simulink model "Microstick_II_CodeReplacementLookup_ExternalMode_R2016b"  (R2016b)
settings: Solver=FixedStepDiscrete  StartTime=0.0  StopTime=inf  FixedStep=0.01  RelTol=1e-3
undefined symbols (not defined in the file or in its folder): A4, B0, B10, B11, B12, Max, MaxPer, ms, P20, P32, P42, P43, Pin, Resol, us
libraries: MCHP_Blockset x10
(part 2 of 2)

== system Microstick_II_CodeReplacementLookup_ExternalMode_R2016b/Cos/Cos Q15 ==
  In2 : Inport
  MCHP_Cos_Q1.15 : Subsystem  TreatAsAtomicUnit=on
  Cos_Out1 : Outport  OutDataTypeStr=fixdt(1,16,14)
  wires:
  In2/1 -> MCHP_Cos_Q1.15/1(In1)
  MCHP_Cos_Q1.15/1(Out1) -> Cos_Out1/1

== system Microstick_II_CodeReplacementLookup_ExternalMode_R2016b/Microstick2 - dsPIC33EP128MC202/1Hz Blinking2 ==
  Delay : Delay  DelayLength=1  InitialCondition=0  SampleTime=.5
  Logical Operator : Logic  Operator=NOT  AllPortsSameDT=off  OutDataTypeStr=boolean
  Rate Transition2 : RateTransition  Deterministic=off  OutPortSampleTime=.05
  Out1 : Outport
  wires:
  Delay/1 -> Logical Operator/1
  Logical Operator/1 -> Delay/1, Rate Transition2/1
  Rate Transition2/1 -> Out1/1

== system Microstick_II_CodeReplacementLookup_ExternalMode_R2016b/Microstick2 - dsPIC33EP128MC202/Open board doc WWW ==

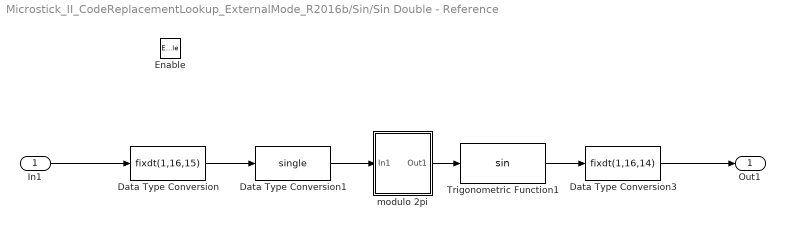
== system Microstick_II_CodeReplacementLookup_ExternalMode_R2016b/Sin/Sin Double - Reference ==
  In1 : Inport
  Enable : EnablePort
  Data Type Conversion : DataTypeConversion  OutDataTypeStr=fixdt(1,16,15)  ConvertRealWorld=Stored Integer (SI)
  Data Type Conversion1 : DataTypeConversion  OutDataTypeStr=single
  Data Type Conversion3 : DataTypeConversion  OutDataTypeStr=fixdt(1,16,14)  RndMeth=Convergent  SaturateOnIntegerOverflow=on
  Trigonometric Function1 : Trigonometry  NumberOfIterations=15
  modulo 2pi : Subsystem
  Out1 : Outport
  wires:
  Data Type Conversion3/1 -> Out1/1
  modulo 2pi/1(Out1) -> Trigonometric Function1/1
  Data Type Conversion1/1 -> modulo 2pi/1(In1)
  Data Type Conversion/1 -> Data Type Conversion1/1
  Trigonometric Function1/1 -> Data Type Conversion3/1
  In1/1 -> Data Type Conversion/1

== system Microstick_II_CodeReplacementLookup_ExternalMode_R2016b/Sin/Sin Q15 ==
  In2 : Inport
  MCHP_Sin_Q1.15 : Subsystem  TreatAsAtomicUnit=on
  Sin_Out1 : Outport  OutDataTypeStr=fixdt(1,16,14)
  wires:
  MCHP_Sin_Q1.15/1(Out1) -> Sin_Out1/1
  In2/1 -> MCHP_Sin_Q1.15/1(In1)

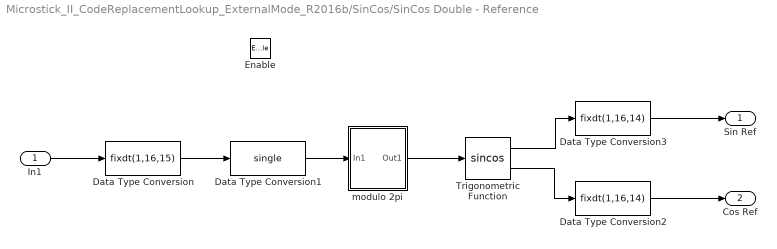
== system Microstick_II_CodeReplacementLookup_ExternalMode_R2016b/SinCos/SinCos Double - Reference ==
  In1 : Inport
  Enable : EnablePort
  Data Type Conversion : DataTypeConversion  OutDataTypeStr=fixdt(1,16,15)  ConvertRealWorld=Stored Integer (SI)
  Data Type Conversion1 : DataTypeConversion  OutDataTypeStr=single
  Data Type Conversion2 : DataTypeConversion  OutDataTypeStr=fixdt(1,16,14)  RndMeth=Convergent  SaturateOnIntegerOverflow=on
  Data Type Conversion3 : DataTypeConversion  OutDataTypeStr=fixdt(1,16,14)  RndMeth=Convergent  SaturateOnIntegerOverflow=on
  Trigonometric Function : Trigonometry  Operator=sincos
  modulo 2pi : Subsystem
  Sin Ref : Outport
  Cos Ref : Outport  Port=2
  wires:
  Data Type Conversion3/1 -> Sin Ref/1
  modulo 2pi/1(Out1) -> Trigonometric Function/1
  Data Type Conversion1/1 -> modulo 2pi/1(In1)
  Data Type Conversion/1 -> Data Type Conversion1/1
  Trigonometric Function/1 -> Data Type Conversion3/1
  In1/1 -> Data Type Conversion/1
  Data Type Conversion2/1 -> Cos Ref/1
  Trigonometric Function/2 -> Data Type Conversion2/1

== system Microstick_II_CodeReplacementLookup_ExternalMode_R2016b/SinCos/SinCos Q15 ==
  In2 : Inport
  MCHP_SinCos_Q1.15 : Subsystem  TreatAsAtomicUnit=on
  Sin_Out : Outport  OutDataTypeStr=fixdt(1,16,14)
  Cos_Out : Outport  Port=2  OutDataTypeStr=fixdt(1,16,14)
  wires:
  MCHP_SinCos_Q1.15/1(Out1) -> Sin_Out/1
  In2/1 -> MCHP_SinCos_Q1.15/1(In1)
  MCHP_SinCos_Q1.15/2(Out2) -> Cos_Out/1

== system Microstick_II_CodeReplacementLookup_ExternalMode_R2016b/Sqrt/ Sqrt Q15 ==
  In1 : Inport
  Sqrt : Sqrt  OutDataTypeStr=fixdt(1,16,15)
  Out1 : Outport
  wires:
  Sqrt/1 -> Out1/1
  In1/1 -> Sqrt/1

== system Microstick_II_CodeReplacementLookup_ExternalMode_R2016b/Sqrt/Sqrt Double - Reference  ==
  In1 : Inport
  Enable : EnablePort
  Data Type Conversion8 : DataTypeConversion  OutDataTypeStr=single
  Sqrt1 : Sqrt  OutDataTypeStr=fixdt(1,16,15)  RndMeth=Convergent
  Out2 : Outport
  wires:
  Sqrt1/1 -> Out2/1
  Data Type Conversion8/1 -> Sqrt1/1
  In1/1 -> Data Type Conversion8/1

== system Microstick_II_CodeReplacementLookup_ExternalMode_R2016b/Atan2/Atan2 Q15/Atan2_Q1.15 ==
  In1 : Inport
  In2 : Inport  Port=2
  Atan2 : Trigonometry  Operator=atan2  ApproximationMethod=CORDIC  NumberOfIterations=15  OutputSignalType=real
  Out1 : Outport
  wires:
  Atan2/1 -> Out1/1
  In1/1 -> Atan2/1
  In2/1 -> Atan2/2

== system Microstick_II_CodeReplacementLookup_ExternalMode_R2016b/Atan2/Double Atan2 - Reference/Simulink_Q1.15 ==
  In1 : Inport
  In2 : Inport  Port=2
  Data Type Conversion1 : DataTypeConversion  OutDataTypeStr=single
  Data Type Conversion3 : DataTypeConversion  OutDataTypeStr=single
  Data Type Conversion4 : DataTypeConversion  OutDataTypeStr=fixdt(1,16,13)  RndMeth=Convergent  SaturateOnIntegerOverflow=on
  Trigonometric Function1 : Trigonometry  Operator=atan2  NumberOfIterations=14  OutputSignalType=real
  Out1 : Outport
  wires:
  In2/1 -> Data Type Conversion3/1
  In1/1 -> Data Type Conversion1/1
  Data Type Conversion1/1 -> Trigonometric Function1/1
  Data Type Conversion3/1 -> Trigonometric Function1/2
  Trigonometric Function1/1 -> Data Type Conversion4/1
  Data Type Conversion4/1 -> Out1/1

== system Microstick_II_CodeReplacementLookup_ExternalMode_R2016b/Cos/Cos Double - Reference/modulo 2pi ==
  In1 : Inport
  Bias : Bias  Bias=pi
  Bias1 : Bias  Bias=-pi
  Constant2 : Constant  Value=2*pi  OutDataTypeStr=single  SampleTime=-1
  Math Function : Math  Operator=mod  SaturateOnIntegerOverflow=on
  Out1 : Outport
  wires:
  Bias1/1 -> Out1/1
  Bias/1 -> Math Function/1
  Constant2/1 -> Math Function/2
  Math Function/1 -> Bias1/1
  In1/1 -> Bias/1

== system Microstick_II_CodeReplacementLookup_ExternalMode_R2016b/Cos/Cos Q15/MCHP_Cos_Q1.15 ==
  In1 : Inport
  Cos : Trigonometry  Operator=cos  ApproximationMethod=CORDIC  NumberOfIterations=16
  Out1 : Outport
  wires:
  In1/1 -> Cos/1
  Cos/1 -> Out1/1

== system Microstick_II_CodeReplacementLookup_ExternalMode_R2016b/Sin/Sin Double - Reference/modulo 2pi ==
  In1 : Inport
  Bias : Bias  Bias=pi
  Bias1 : Bias  Bias=-pi
  Constant2 : Constant  Value=2*pi  OutDataTypeStr=single  SampleTime=-1
  Math Function : Math  Operator=mod  SaturateOnIntegerOverflow=on
  Out1 : Outport
  wires:
  In1/1 -> Bias/1
  Math Function/1 -> Bias1/1
  Constant2/1 -> Math Function/2
  Bias/1 -> Math Function/1
  Bias1/1 -> Out1/1

== system Microstick_II_CodeReplacementLookup_ExternalMode_R2016b/Sin/Sin Q15/MCHP_Sin_Q1.15 ==
  In1 : Inport
  Sin : Trigonometry  ApproximationMethod=CORDIC  NumberOfIterations=16
  Out1 : Outport
  wires:
  Sin/1 -> Out1/1
  In1/1 -> Sin/1

== system Microstick_II_CodeReplacementLookup_ExternalMode_R2016b/SinCos/SinCos Double - Reference/modulo 2pi ==
  In1 : Inport
  Bias : Bias  Bias=pi
  Bias1 : Bias  Bias=-pi
  Constant2 : Constant  Value=2*pi  OutDataTypeStr=single  SampleTime=-1
  Math Function : Math  Operator=mod  SaturateOnIntegerOverflow=on
  Out1 : Outport
  wires:
  In1/1 -> Bias/1
  Math Function/1 -> Bias1/1
  Constant2/1 -> Math Function/2
  Bias/1 -> Math Function/1
  Bias1/1 -> Out1/1

== system Microstick_II_CodeReplacementLookup_ExternalMode_R2016b/SinCos/SinCos Q15/MCHP_SinCos_Q1.15 ==
  In1 : Inport
  SinCos : Trigonometry  Operator=sincos  ApproximationMethod=CORDIC  NumberOfIterations=16
  Out1 : Outport
  Out2 : Outport  Port=2
  wires:
  SinCos/1 -> Out1/1
  In1/1 -> SinCos/1
  SinCos/2 -> Out2/1
